simulink model "TrafficMoore"  (R2020b)
settings: Solver=VariableStepAuto  StartTime=0.0  StopTime=10.0  RelTol=1e-3
settings Model: Creator=Sourav Kumar  LastModifiedBy=Sourav Kumar

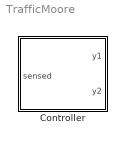
== system TrafficMoore ==
  Controller : Stateflow chart  TreatAsAtomicUnit=on

== stateflow chart TrafficMoore/Controller ==
  settings: stateMachineType=MOORE_MACHINE  initializeOutput=1
  state Stop
    y1=Red;
    y2=Green;
  state StopForTraffic
    y1=Red;
    y2=Green;
  state StopToGo
    y1=Red;
    y2=Yellow;
  state GoToStop
    y1=Yellow;
    y2=Red;
  state Go
    y1=Green;
    y2=Red;
  (default) -> Stop
  Stop -> StopForTraffic : after(20,tick)
  StopForTraffic -> StopToGo : [sensed]
  GoToStop -> Stop : after(5,tick)
  StopToGo -> Go : after(5,tick)
  Go -> GoToStop : after(12,tick)
  data: y1 output; y2 output; Red constant double =1; Yellow constant double =2; Green constant double =3; sensed input
